simulink subsystem "State_Interpreter"  (R2023b)
settings: Solver=VariableStepAuto  StartTime=0.0  StopTime=10.0  RelTol=1e-3
undefined symbols (not defined in the file): All_Autos, All_Autos_Sizes, Auto_Design_Path, Auto_Intake_Velocity, Auto_Start_Time, Auto_Start_Velocity
libraries: simulink x5
settings Model: Creator=FIRSTMentor  LastModifiedBy=ander

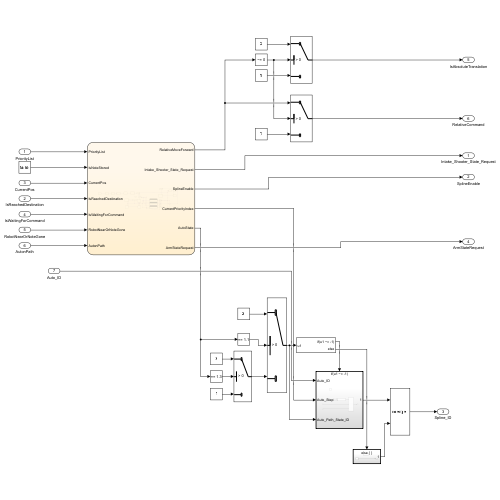
[thumbnail: Simulink's stored preview of the top-level diagram]
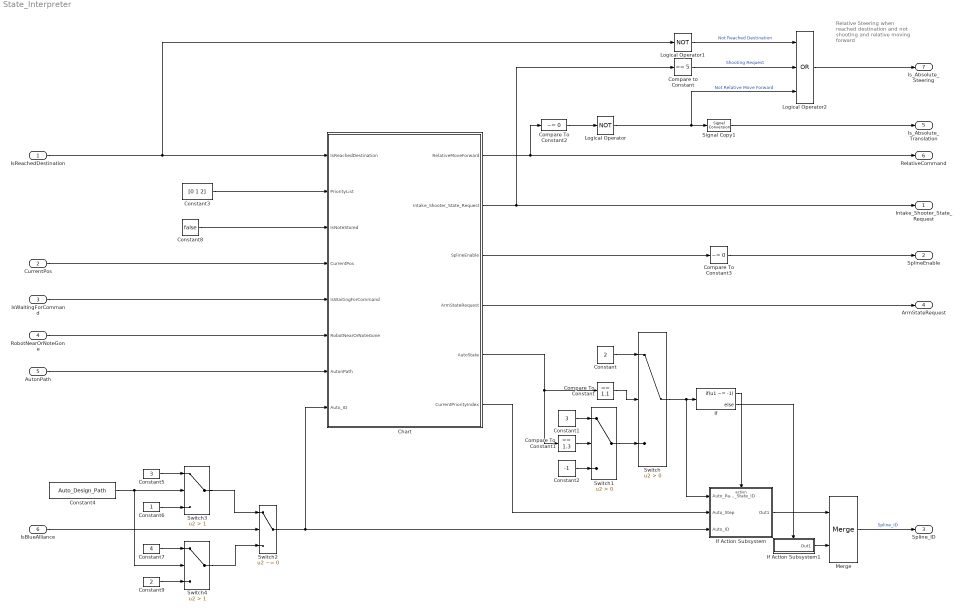
== system State_Interpreter ==
  note: Relative Steering when
      | reached destination and
      | not shooting and
      | relative moving forward
  IsReachedDestination : Inport  OutDataTypeStr=boolean  PortDimensions=1
  CurrentPos : Inport  Port=2
  IsWaitingForCommand : Inport  Port=3  OutDataTypeStr=boolean  PortDimensions=1
  RobotNearOrNoteGone : Inport  Port=4
  AutonPath : Inport  Port=5
  IsBlueAlliance : Inport  Port=6
  Chart : Stateflow chart  TreatAsAtomicUnit=on
      settings: PortSchema="{\"entries\":[{\"content\":{\"sides\":[{\"content\":{\"connectorIds\":[\"In4\",\"In1\",\"In2\",\"In3\",\"In5\",\"In6\",\"In7\",\"In8\"]},\"type\":\"ConnectorPlacement.EquallySpacedRectSide\",\"uuid\":\"1d1cc9bd-66ff-45b7-9349-9ce48823472f\"},{\"content\":{\"connectorIds\":[\"Out6\",\"Out1\",\"Out2\",\"Out5\",\"Out4\",\"Out3\"],\"side\":\"RIGHT\"},\"type\":\"ConnectorPlacement.EquallySpacedRectSide\",\"uuid\":\"1aa3abc4-7068-49fd-b3da-164567a4afb0\"},{\"content\":{\"side\":\"TOP\"},\"type\":\"ConnectorPlacement.EquallySpacedRectSide\",\"uuid\":\"e686b79c-9dcc-4208-9677-ddd16b311e30\"}]},\"type\":\"ConnectorPlacement.EquallySpacedConnector\",\"uuid\":\"76a55cdc-47cf-48fb-bbe6-7150d837bb59\"}],\"packageUris\":[\"http://schema.mathworks.com/mf0/Connector/R2020b\"],\"version\":\"1.0\"}"
  Compare To Constant : simulink/Logic and Bit Operations/Compare To Constant  relop===  const=1.1  OutDataTypeStr=boolean
  Compare To Constant1 : simulink/Logic and Bit Operations/Compare To Constant  relop===  const=1.3  OutDataTypeStr=boolean
  Compare To Constant2 : simulink/Logic and Bit Operations/Compare To Constant  relop=~=  const=0  OutDataTypeStr=boolean
  Compare To Constant3 : simulink/Logic and Bit Operations/Compare To Constant  relop=~=  const=0  OutDataTypeStr=boolean
  Compare to Constant : simulink/Logic and Bit Operations/Compare To Constant  relop===  const=5  OutDataTypeStr=boolean
  Constant : Constant  Value=2
  Constant1 : Constant  Value=3
  Constant2 : Constant  Value=-1
  Constant3 : Constant  Value=[0 1 2]
  Constant4 : Constant  Value=Auto_Design_Path
  Constant5 : Constant  Value=3
  Constant6 : Constant
  Constant7 : Constant  Value=4
  Constant8 : Constant  Value=false
  Constant9 : Constant  Value=2
  If : If  IfExpression=u1 ~= -1
  If Action Subsystem : Subsystem  TreatAsAtomicUnit=on
  If Action Subsystem1 : Subsystem  TreatAsAtomicUnit=on
  Logical Operator : Logic  Operator=NOT  AllPortsSameDT=off  OutDataTypeStr=boolean
  Logical Operator1 : Logic  Operator=NOT  AllPortsSameDT=off  OutDataTypeStr=boolean
  Logical Operator2 : Logic  Operator=OR  Inputs=3  AllPortsSameDT=off  OutDataTypeStr=boolean
  Merge : Merge
  Signal Copy1 : SignalConversion  OverrideOpt=off
  Switch : Switch  Criteria=u2 > Threshold  SaturateOnIntegerOverflow=off  InputSameDT=off
  Switch1 : Switch  Criteria=u2 > Threshold  SaturateOnIntegerOverflow=off  InputSameDT=off
  Switch2 : Switch  Criteria=u2 ~= 0  SaturateOnIntegerOverflow=off  InputSameDT=off
  Switch3 : Switch  Criteria=u2 > Threshold  Threshold=1  SaturateOnIntegerOverflow=off  InputSameDT=off
  Switch4 : Switch  Criteria=u2 > Threshold  Threshold=1  SaturateOnIntegerOverflow=off  InputSameDT=off
  Intake_Shooter_State_Request : Outport
  SplineEnable : Outport  Port=2
  Spline_ID : Outport  Port=3
  ArmStateRequest : Outport  Port=4
  Is_Absolute_Translation : Outport  Port=5
  RelativeCommand : Outport  Port=6
  Is_Absolute_Steering : Outport  Port=7
  wires:
  Constant7/1 -> Switch4/1
  Constant4/1 -> Switch4/2, Switch3/2
  Constant9/1 -> Switch4/3
  Constant6/1 -> Switch3/3
  Constant5/1 -> Switch3/1
  Switch4/1 -> Switch2/3
  Switch3/1 -> Switch2/1
  IsBlueAlliance/1 -> Switch2/2
  Logical Operator/1 -> Signal Copy1/1, Logical Operator2/3  "Not Relative Move Forward"
  Chart/6(RelativeMoveForward) -> Compare To Constant2/1, RelativeCommand/1
  Compare To Constant2/1 -> Logical Operator/1
  Chart/5(ArmStateRequest) -> ArmStateRequest/1
  Merge/1 -> Spline_ID/1  "Spline_ID"
  Switch/1 -> If Action Subsystem/1(Auto_Path_State_ID), If/1
  Constant/1 -> Switch/1
  Constant1/1 -> Switch1/1
  Constant2/1 -> Switch1/3
  Compare To Constant1/1 -> Switch1/2
  Compare To Constant/1 -> Switch/2
  Switch1/1 -> Switch/3
  Chart/4(AutoState) -> Compare To Constant1/1, Compare To Constant/1
  Chart/2(SplineEnable) -> Compare To Constant3/1
  Chart/1(Intake_Shooter_State_Request) -> Compare to Constant/1, Intake_Shooter_State_Request/1
  AutonPath/1 -> Chart/7(AutonPath)
  RobotNearOrNoteGone/1 -> Chart/6(RobotNearOrNoteGone)
  IsWaitingForCommand/1 -> Chart/5(IsWaitingForCommand)
  IsReachedDestination/1 -> Logical Operator1/1, Chart/4(IsReachedDestination)
  CurrentPos/1 -> Chart/3(CurrentPos)
  Constant8/1 -> Chart/2(IsNoteStored)
  Constant3/1 -> Chart/1(PriorityList)
  Chart/3(CurrentPriorityIndex) -> If Action Subsystem/2(Auto_Step)
  Switch2/1 -> If Action Subsystem/3(Auto_ID), Chart/8(Auto_ID)
  If Action Subsystem1/1(Out1) -> Merge/2
  If Action Subsystem/1(Out1) -> Merge/1
  If/1 -> If Action Subsystem/Action
  If/2 -> If Action Subsystem1/Action
  Logical Operator1/1 -> Logical Operator2/1  "Not Reached Destination"
  Compare to Constant/1 -> Logical Operator2/2  "Shooting Request"
  Logical Operator2/1 -> Is_Absolute_Steering/1
  Signal Copy1/1 -> Is_Absolute_Translation/1
  Compare To Constant3/1 -> SplineEnable/1

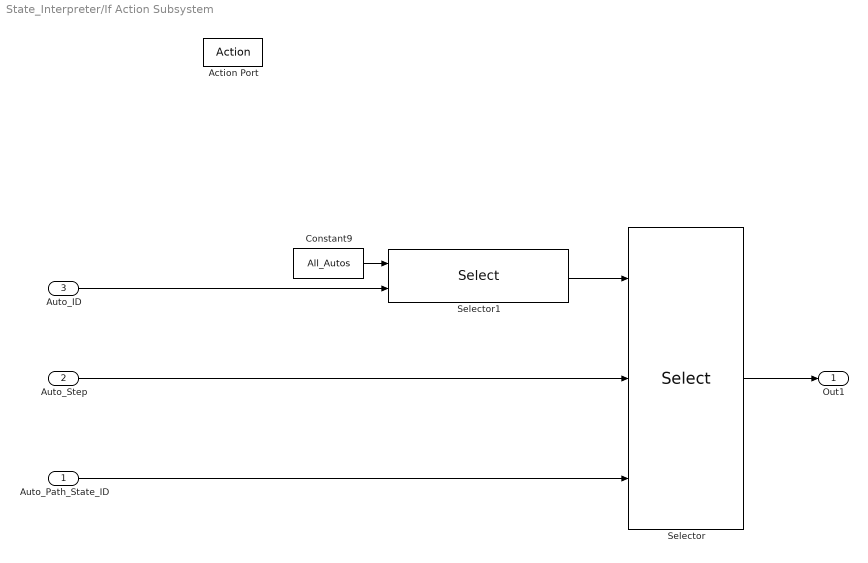
== system State_Interpreter/If Action Subsystem ==
  Auto_Path_State_ID : Inport
  Auto_Step : Inport  Port=2
  Auto_ID : Inport  Port=3
  Action Port : ActionPort
  Constant9 : Constant  Value=All_Autos  VectorParams1D=off
  Selector : Selector  NumberOfDimensions=2  InputPortWidth=3  IndexOptions=Index vector (port),Index vector (port)  Indices=[1 3],1  OutputSizes=1,1
  Selector1 : Selector  NumberOfDimensions=3  InputPortWidth=3  IndexOptions=Select all,Select all,Index vector (port)  Indices=[1 3],1,1  OutputSizes=1,1,1
  Out1 : Outport
  wires:
  Auto_ID/1 -> Selector1/2
  Selector1/1 -> Selector/1
  Constant9/1 -> Selector1/1
  Auto_Step/1 -> Selector/2
  Auto_Path_State_ID/1 -> Selector/3
  Selector/1 -> Out1/1

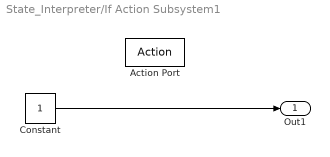
== system State_Interpreter/If Action Subsystem1 ==
  Action Port : ActionPort
  Constant : Constant
  Out1 : Outport
  wires:
  Constant/1 -> Out1/1

== stateflow chart State_Interpreter/Chart ==
  state PathToPickUpWODetec
    en:
    AutoState = 1.1;
    SplineEnable = 1;
    Intake_Shooter_State_Request = 1;
    Timer = t_sample;
    du:
    Timer = Timer + t_sample;
  state ShootWODetec
    en:
    AutoState = 1.0;
    SplineEnable = 0;
    RelativeMoveForward = 0;
    Intake_Shooter_State_Request = 5;
    Timer = t_sample;
    du:
    Timer = Timer + t_sample;
    ex:
    Intake_Shooter_State_Request = 0;
  state MoveArms_and_MoveForward
    en:
    ArmStateRequest = 1;
    SplineEnable = 0;
    RelativeMoveForward = Auto_Start_Velocity;
    Timer = t_sample;
    du:
    Timer = Timer + t_sample;
  state ShootNote
    en:
    Timer = t_sample;
    Intake_Shooter_State_Request = 5;
    du:
    Timer = Timer + t_sample;
    ex:
    Intake_Shooter_State_Request = 0;
  state Move_To_Shoot
    en:
    Timer = t_sample;
    RelativeMoveForward = .5;
    du:
    Timer = Timer + t_sample;
    ex:
    RelativeMoveForward = 0;
  state AngleArms
    en:
    ArmStateRequest = 1;
    Timer = t_sample;
    du:
    Timer = Timer + t_sample
  state ShootAgain
    en:
    Timer = t_sample;
    Intake_Shooter_State_Request = 5;
    du:
    Timer = Timer + t_sample;
    ex:
    Intake_Shooter_State_Request = 0;
  state DriveBack
    en:
    Timer = t_sample;
    RelativeMoveForward = -1;
    du:
    Timer = Timer + t_sample;
    ex:
    RelativeMoveForward = 0;
  state DriveOut
    en:
    Timer = t_sample;
    Intake_Shooter_State_Request = 1;
    RelativeMoveForward = .5;
    du:
    Timer = Timer + t_sample;
    ex:
    Intake_Shooter_State_Request = 0;
    RelativeMoveForward = 0;
  state Stop
  state RunIntake1
    en:
    AutoState = 1.2;
    SplineEnable = 0;
    RelativeMoveForward = Auto_Intake_Velocity;
    Timer = t_sample;
    du:
    Timer = Timer + t_sample;
    ex:
    RelativeMoveForward = 0;
  state Reset_SPF
    en:
    SplineEnable = 0;
  state PathToShootWODetec
    en:
    AutoState = 1.3;
    SplineEnable = 1;
    Intake_Shooter_State_Request = 6;
  state PathPicker
    en:
    CloseNoteCounter = 0;
    RelativeMoveForward = 0;
  state Auto Detection [group]
    path will be path
    10
  state CheckForRobotOrNote
    en:
    Intake_Shooter_State_Request = 0;
    SplineEnable = 0;
    Timer = t_sample;
    du:
    Timer = Timer + t_sample;
    ex:
    CurrentPriorityIndex = CurrentPriorityIndex + 1;
  state Note6
    state Shoot1
      en:
      Intake_Shooter_State_Request = 1;
      SplineEnable = 0;
      Timer = t_sample;
      du:
      Timer = Timer + t_sample;
      ex:
      Intake_Shooter_State_Request = 0;
    state PathToShoot1
      en:
      SplineEnable = 1;
      CloseNoteCounter = CloseNoteCounter + 1;
      ex:
      SplineEnable = 0;
    174 -> Note6.PathToShoot1
    Note6.PathToShoot1 -> Note6.Shoot1
    Note6.Shoot1 -> 179 : [IsWaitingForCommand]
  state Shoot
    en:
    Intake_Shooter_State_Request = 1;
    SplineEnable = 0;
    Timer = t_sample;
    du:
    Timer = Timer + t_sample;
    ex:
    Intake_Shooter_State_Request = 0;
  state PathToPickUp
    en:
    SplineEnable = 1;
    ex:
    SplineEnable = 0;
  state Note6_trans
  state Note7
    state Shoot1
      en:
      Intake_Shooter_State_Request = 1;
      SplineEnable = 0;
      Timer = t_sample;
      du:
      Timer = Timer + t_sample;
      ex:
      Intake_Shooter_State_Request = 0;
    state PathToShoot1
      en:
      SplineEnable = 1;
      CloseNoteCounter = CloseNoteCounter + 1;
      ex:
      SplineEnable = 0;
    Note7.Shoot1 -> 186 : [IsWaitingForCommand]
    187 -> Note7.PathToShoot1
    Note7.PathToShoot1 -> Note7.Shoot1
  state Note7_trans
  state End
  state RunIntake
    en:
    SplineEnable = 1;
    Intake_Shooter_State_Request = 1;
    ex:
    Intake_Shooter_State_Request = 0;
    SplineEnable = 0;
  state PathToShoot
    en:
    SplineEnable = 1;
    ex:
    SplineEnable = 0;
  state Note8
    state Shoot1
      en:
      Intake_Shooter_State_Request = 1;
      SplineEnable = 0;
      Timer = t_sample;
      du:
      Timer = Timer + t_sample;
      ex:
      Intake_Shooter_State_Request = 0;
    state PathToShoot1
      en:
      SplineEnable = 1;
      CloseNoteCounter = CloseNoteCounter + 1;
      ex:
      SplineEnable = 0;
    197 -> Note8.PathToShoot1
    Note8.PathToShoot1 -> Note8.Shoot1
    Note8.Shoot1 -> 196 : [IsWaitingForCommand]
  state Note8_trans
  ShootWODetec -> PathToPickUpWODetec [order 2] : [IsWaitingForCommand || Timer > 3]{CurrentPriorityIndex = CurrentPriorityIndex + 1;}
  ShootWODetec -> (junction 515) [order 1] : [(IsWaitingForCommand || Timer > 4) && CurrentPriorityIndex == All_Autos_Sizes(Auto_ID)]
  (junction 515) -> (junction 518)
  PathToPickUpWODetec -> RunIntake1 [order 2] : [IsReachedDestination]
  PathToPickUpWODetec -> Reset_SPF [order 1] : [IsWaitingForCommand && ...
      | Timer >= 0.06]
  MoveArms_and_MoveForward -> ShootWODetec : [Timer > Auto_Start_Time]
  (junction 534) -> MoveArms_and_MoveForward
  (junction 524) -> (junction 534)
  PathToShootWODetec -> ShootWODetec : % Do not wait for reaching destination
      | % for first two Auto designs
      | % [Auto_ID <= 2 || ...
      | [IsReachedDestination]
  (junction 522) -> (junction 524)
  (junction 482) -> (junction 524)
  PathPicker -> (junction 522) [order 1] : [AutonPath == 4]
  ShootNote -> DriveOut : [IsWaitingForCommand || Timer > 10]
  AngleArms -> Move_To_Shoot : [Timer > 1]
  DriveBack -> ShootAgain : [Timer > 2.5]
  DriveOut -> DriveBack : [Timer > 5]
  Move_To_Shoot -> ShootNote : [Timer > 1.5]
  ShootAgain -> Stop : [IsWaitingForCommand || Timer > 10]
  PathPicker -> AngleArms [order 6] : [AutonPath == 5]
  PathPicker -> (junction 423) [order 5] : [AutonPath == 3]
  Reset_SPF -> PathToShootWODetec
  (junction 423) -> (junction 216)
  PathPicker -> (junction 422) [order 4] : [AutonPath == 2]
  (junction 422) -> (junction 214)
  PathPicker -> (junction 267) [order 3] : [AutonPath == 1]
  (junction 267) -> (junction 212)
  RunIntake1 -> PathToShootWODetec : [IsWaitingForCommand || Timer >= 4]
  PathPicker -> Shoot [order 2] : [AutonPath == 10]
  (default) -> PathPicker
  (junction 428) -> (junction 482)
  Shoot -> PathToPickUp [order 1] : [PriorityList(CurrentPriorityIndex) < 6]
  PathToPickUp -> CheckForRobotOrNote [order 1] : [Timer  < 16]
  Note6_trans -> (junction 125) [order 5] : [~IsWaitingForCommand]
  (junction 125) -> End
  180 -> Note6_trans
  CheckForRobotOrNote -> PathToPickUp [order 3] : [PriorityList(CurrentPriorityIndex) < 6 && RobotNearOrNoteGone]
  (junction 90) -> (junction 212)
  (junction 212) -> 175
  (junction 229) -> (junction 212)
  (junction 89) -> (junction 90) [order 1] : [PriorityList(CurrentPriorityIndex) == 6 || (CurrentPos == (1) || (2))]
  Note6_trans -> (junction 428) [order 4] : [CloseNoteCounter == 3 && ( AutonPath == 3 || AutonPath == 2)]
  Note6_trans -> (junction 220) [order 3] : [~IsReachedDestination]
  Note7_trans -> Note6_trans [order 2] : [CloseNoteCounter == 2]
  Note6_trans -> Note7_trans [order 2] : [CloseNoteCounter == 1]
  Note8_trans -> Note6_trans [order 2] : [CloseNoteCounter == 2]
  Note6_trans -> Note8_trans [order 1] : [CloseNoteCounter == 2]
  (junction 430) -> (junction 428)
  PathToPickUp -> (junction 50) [order 2] : [Timer  < 16]
  CheckForRobotOrNote -> (junction 49) [order 2] : [PriorityList(CurrentPriorityIndex) > 5 && RobotNearOrNoteGone]
  CheckForRobotOrNote -> RunIntake [order 1] : [~RobotNearOrNoteGone]
  (junction 220) -> (junction 229)
  PathToShoot -> Shoot [order 1] : [PriorityList(CurrentPriorityIndex) < 6]
  Shoot -> (junction 51) [order 2] : [PriorityList(CurrentPriorityIndex) > 5]
  184 -> Note7_trans
  Note7_trans -> End [order 4] : [~IsWaitingForCommand]
  (junction 518) -> End
  (junction 89) -> (junction 214) [order 3] : [PriorityList(CurrentPriorityIndex) == 7 || CurrentPos == 3]
  (junction 214) -> 183
  (junction 51) -> (junction 89)
  (junction 49) -> (junction 50) : [Timer  < 16]
  (junction 50) -> (junction 51)
  (junction 89) -> (junction 92) [order 2] : [PriorityList(CurrentPriorityIndex) == 8 || (CurrentPos == (4) || (5) )]
  (junction 226) -> (junction 214)
  RunIntake -> (junction 49) [order 2] : [~IsNoteStored &&PriorityList(CurrentPriorityIndex) < 6 ]
  PathToShoot -> (junction 51) [order 2] : [PriorityList(CurrentPriorityIndex) > 5]
  Note7_trans -> (junction 221) [order 3] : [~IsReachedDestination]
  Note8_trans -> Note7_trans [order 1] : [CloseNoteCounter == 1]
  Note7_trans -> Note8_trans [order 1] : [CloseNoteCounter == 1]
  (junction 128) -> End
  (junction 221) -> (junction 226)
  RunIntake -> PathToShoot [order 1] : [IsNoteStored]
  194 -> Note8_trans
  Note8_trans -> (junction 128) [order 5] : [~IsWaitingForCommand]
  (junction 92) -> (junction 216)
  (junction 216) -> 193
  (junction 223) -> (junction 216)
  Note8_trans -> (junction 430) [order 4] : [CloseNoteCounter == 3 && AutonPath == 1]
  Note8_trans -> (junction 222) [order 3] : [~IsReachedDestination]
  (junction 222) -> (junction 223)
  data: PriorityList input; Intake_Shooter_State_Request output; IsNoteStored input; CurrentPos input; SplineEnable output double; IsReachedDestination input boolean size=1; CurrentPriorityIndex output =0; Timer local; t_sample constant double =t_sample; IsWaitingForCommand input; RobotNearOrNoteGone input; CloseNoteCounter local; AutonPath input; AutoState output; ArmStateRequest output =0; RelativeMoveForward output; All_Autos_Sizes parameter; Auto_Start_Velocity parameter; Auto_Intake_Velocity parameter; Auto_Start_Time parameter; Auto_ID input
